simulink subsystem "Day1_Scenario_2"  (R2024a)
settings: Solver=VariableStepAuto  StartTime=0.0  StopTime=10.0  RelTol=1e-3
libraries: CarMaker4SL x2
settings Model: Creator=junhyung.cha  LastModifiedBy=pc

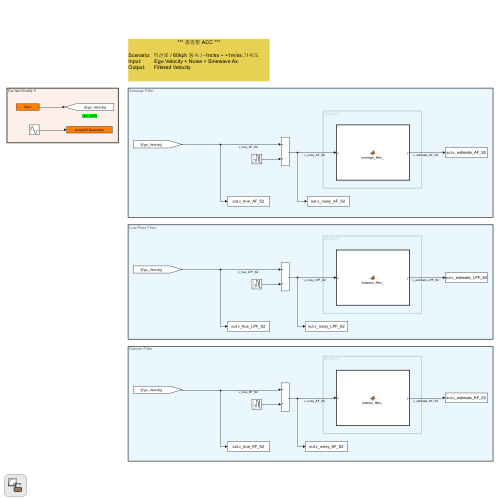
[thumbnail: Simulink's stored preview of the top-level diagram]
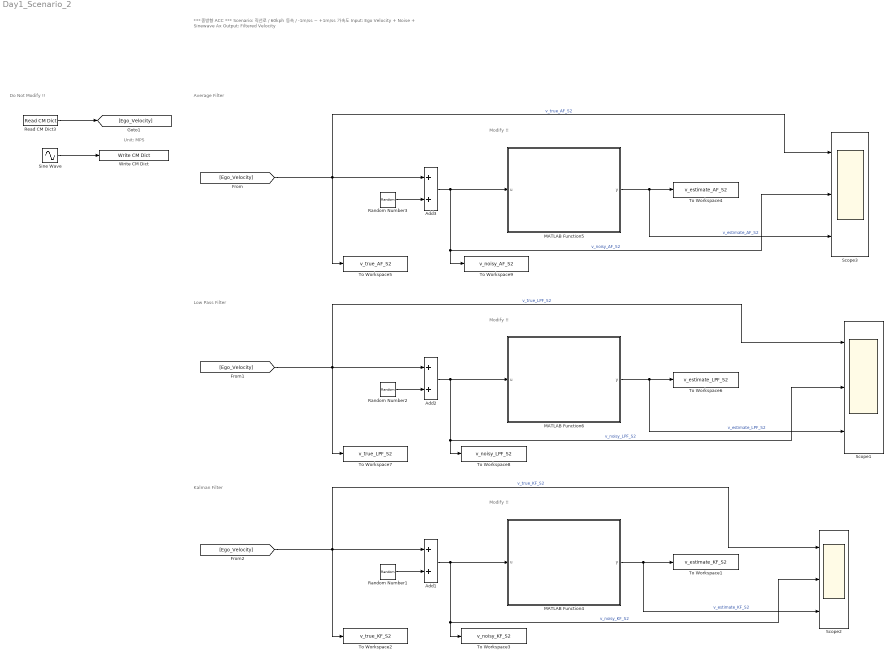
== system Day1_Scenario_2 ==
  note: Do Not Modify !!
  note: Low Pass Filter
  note: Average Filter
  note: Modify !!
  note: Modify !!
  note: Kalman Filter
  note: Modify !!
  note: *** 종방향 ACC ***
      |
      | Scenario: 직선로 / 60kph 등속 / -1m/ss ~ +1m/ss 가속도
      | Input: Ego Velocity + Noise + Sinewave Ax
      | Output: Filtered Velocity
  note: Unit: MPS
  Add1 : Sum
  Add2 : Sum
  Add3 : Sum
  MATLAB Function4 : MATLAB Function  TreatAsAtomicUnit=on
  MATLAB Function5 : MATLAB Function  TreatAsAtomicUnit=on
  MATLAB Function6 : MATLAB Function  TreatAsAtomicUnit=on
  Random Number1 : RandomNumber
  Random Number2 : RandomNumber
  Random Number3 : RandomNumber
  Read CM Dict3 : CarMaker4SL/Read CM Dict  xname=Car.v  xsync=off  xstime=Inherited
  Scope1 : Scope  NumInputPorts=3
  Scope2 : Scope  NumInputPorts=3
  Scope3 : Scope  NumInputPorts=3
  Sine Wave : Sin
  To Workspace1 : ToWorkspace  VariableName=v_estimate_KF_S2  SaveFormat=Timeseries  SampleTime=-1
  To Workspace2 : ToWorkspace  VariableName=v_true_KF_S2  SaveFormat=Timeseries  SampleTime=-1
  To Workspace3 : ToWorkspace  VariableName=v_noisy_KF_S2  SaveFormat=Timeseries  SampleTime=-1
  To Workspace4 : ToWorkspace  VariableName=v_estimate_AF_S2  SaveFormat=Timeseries  SampleTime=-1
  To Workspace5 : ToWorkspace  VariableName=v_true_AF_S2  SaveFormat=Timeseries  SampleTime=-1
  To Workspace6 : ToWorkspace  VariableName=v_estimate_LPF_S2  SaveFormat=Timeseries  SampleTime=-1
  To Workspace7 : ToWorkspace  VariableName=v_true_LPF_S2  SaveFormat=Timeseries  SampleTime=-1
  To Workspace8 : ToWorkspace  VariableName=v_noisy_LPF_S2  SaveFormat=Timeseries  SampleTime=-1
  To Workspace9 : ToWorkspace  VariableName=v_noisy_AF_S2  SaveFormat=Timeseries  SampleTime=-1
  Write CM Dict : CarMaker4SL/Write CM Dict  xname=AccelCtrl.DesiredAx  xsync=off
  wires:
  Sine Wave/1 -> Write CM Dict/1
  Random Number3/1 -> Add3/2
  Add3/1 -> To Workspace9/1, Scope3/2, MATLAB Function5/1(u)  "v_noisy_AF_S2"
  Add2/1 -> MATLAB Function6/1(u), To Workspace8/1, Scope1/2  "v_noisy_LPF_S2"
  [Ego_Velocity] -> Add2/1, To Workspace7/1, Scope1/1  "v_true_LPF_S2"
  MATLAB Function6/1(y) -> To Workspace6/1, Scope1/3  "v_estimate_LPF_S2"
  Random Number2/1 -> Add2/2
  MATLAB Function5/1(y) -> To Workspace4/1, Scope3/3  "v_estimate_AF_S2"
  Add1/1 -> To Workspace3/1, Scope2/2, MATLAB Function4/1(u)  "v_noisy_KF_S2"
  [Ego_Velocity] -> Add1/1, To Workspace2/1, Scope2/1  "v_true_KF_S2"
  MATLAB Function4/1(y) -> To Workspace1/1, Scope2/3  "v_estimate_KF_S2"
  [Ego_Velocity] -> Add3/1, To Workspace5/1, Scope3/1  "v_true_AF_S2"
  Random Number1/1 -> Add1/2
  Read CM Dict3/1 -> [Ego_Velocity]

== matlab function Day1_Scenario_2/MATLAB Function5 ==
  settings: updateMethod=DISCRETE  sampleTime=0.05
  data: u input; y output
function y = average_filter_(u)
%#codegen

    % 윈도우 크기 정의
    N = 20;

    % persistent 변수 선언 (상태 저장용)
    persistent buffer index count

    if isempty(buffer)
        buffer = zeros(1, N);
        index = 1;
        count = 0;
    end

    % 새로운 입력 저장
    buffer(index) = u;
    index = index + 1;

    % 인덱스 순환
    if index > N
        index = 1;
    end

    % 유효한 샘플 수 갱신
    if count < N
        count = count + 1;
    end

    % 평균 계산
    y = sum(buffer) / count;
    
end

== matlab function Day1_Scenario_2/MATLAB Function6 ==
  settings: updateMethod=DISCRETE  sampleTime=0.05
  data: u input; y output
function y = average_filter_(u)
%#codegen

    % 필터 계수
    alpha = 0.1;

    % 이전 출력값 저장용
    persistent y_prev

    % 초기화
    if isempty(y_prev)
        y_prev = u;
    end

    % 1차 저역통과 필터 적용
    y = alpha * u + (1 - alpha) * y_prev;

    % 현재 출력값을 다음 반복을 위한 이전값으로 저장
    y_prev = y;
end

== matlab function Day1_Scenario_2/MATLAB Function4 ==
  settings: updateMethod=DISCRETE  sampleTime=0.05
  data: u input; y output
function y = average_filter_(u)
% Basic 1D Kalman Filter implementation
% Input: u - measurement (e.g., sensor value)
% Output: y - estimated true value (filtered)

    %#codegen

    % System parameters
    A = 1;
    B = 0;
    C = 1;
    Q = 0.1;  % Process noise covariance
    R = 4;   % Measurement noise covariance

    persistent x_hat P

    if isempty(x_hat)
        x_hat = u;  % Initialize with first measurement
        P = 100;    % Large initial uncertainty
    end

    %------------------ Prediction ------------------%
    x_pred = A * x_hat + B * u;
    P_pred = A * P * A' + Q;

    %------------------ Correction ------------------%
    y_pred = C * x_pred;
    K = P_pred * C' / (C * P_pred * C' + R);
    x_hat = x_pred + K * (u - y_pred);
    P = (1 - K * C) * P_pred;

    % Output the filtered estimate
    y = x_hat;
end
